simulink model "task_1"  (R2023a)
settings: Solver=VariableStepAuto  StartTime=0.0  StopTime=70  RelTol=1e-3  EnableMultiTasking=on
model workspace (MAT data in the model file):
  Tp = 1
  u_liner = 1
settings Model: Creator=Laptop  LastModifiedBy=denys
settings SolverCC: AlgebraicLoopSolver=TrustRegion
settings DataIOCC: ReturnWorkspaceOutputs=off
settings OptimizationCC: LifeSpan=inf
settings DebuggingCC: UnconnectedInputMsg=warning  UnconnectedOutputMsg=warning  UnconnectedLineMsg=warning  SFUnexpectedBacktrackingDiag=warning  SFNoUnconditionalDefaultTransitionDiag=warning  ArithmeticOperatorsInVariantConditions=warning
settings ModelReferenceCC: EnableRefExpFcnMdlSchedulingChecks=on
settings SFSimCC: SimUseLocalCustomCode=off  CustomCodeUndefinedFunction=UseInterfaceOnly
settings RTWCC: RTWUseLocalCustomCode=off
settings CodeAppCC: StateflowObjectComments=on
settings GRTTargetCC: TargetLangStandard=C89/C90 (ANSI)
settings ConfigComp: CovMetricSettings=dw  CovSaveCumulativeToWorkspaceVar=on  CovSaveSingleToWorkspaceVar=on  CovExternalEMLEnable=off

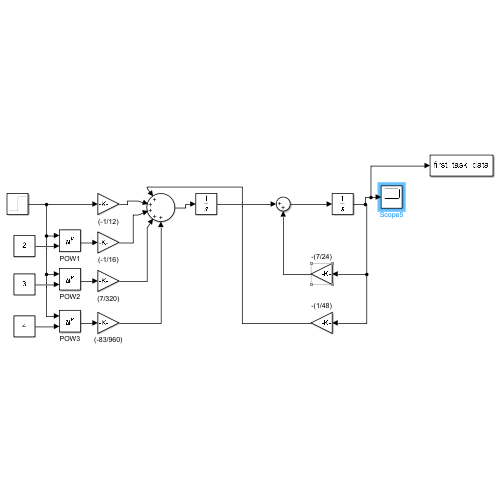
[thumbnail: Simulink's stored preview of the top-level diagram]
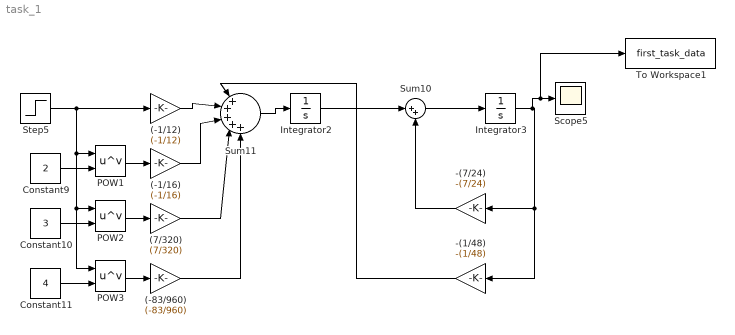
== system task_1 ==
  (-1/12) : Gain  Gain=(-1/12)
  (-1/16) : Gain  Gain=(-1/16)
  (-83/960) : Gain  Gain=(-83/960)
  (7/320) : Gain  Gain=(7/320)
  -(1/48) : Gain  Gain=-(1/48)
  -(7/24) : Gain  Gain=-(7/24)
  Constant10 : Constant  Value=3
  Constant11 : Constant  Value=4
  Constant9 : Constant  Value=2
  Integrator2 : Integrator
  Integrator3 : Integrator
  POW1 : Math  Operator=pow
  POW2 : Math  Operator=pow
  POW3 : Math  Operator=pow
  Scope5 : Scope
  Step5 : Step  SampleTime=0
  Sum10 : Sum  Inputs=|++
  Sum11 : Sum  Inputs=|+++++
  To Workspace1 : ToWorkspace  VariableName=first_task_data  SaveFormat=Timeseries  SampleTime=-1
  wires:
  Constant9/1 -> POW1/2
  POW1/1 -> (-1/16)/1
  (-1/16)/1 -> Sum11/3
  -(7/24)/1 -> Sum10/2
  Sum10/1 -> Integrator3/1
  Constant11/1 -> POW3/2
  (-83/960)/1 -> Sum11/5
  POW2/1 -> (7/320)/1
  Sum11/1 -> Integrator2/1
  Constant10/1 -> POW2/2
  Integrator3/1 -> To Workspace1/1, Scope5/1, -(1/48)/1, -(7/24)/1
  (-1/12)/1 -> Sum11/2
  (7/320)/1 -> Sum11/4
  POW3/1 -> (-83/960)/1
  Step5/1 -> POW3/1, POW2/1, POW1/1, (-1/12)/1
  -(1/48)/1 -> Sum11/1
  Integrator2/1 -> Sum10/1
